simulink model "SVPWM"  (R2019a)
settings: Solver=FixedStepAuto  StartTime=0.0  StopTime=.1  FixedStep=1e-6  RelTol=1e-3
libraries: powerlib x8
settings Model: Creator=sange  LastModifiedBy=sange

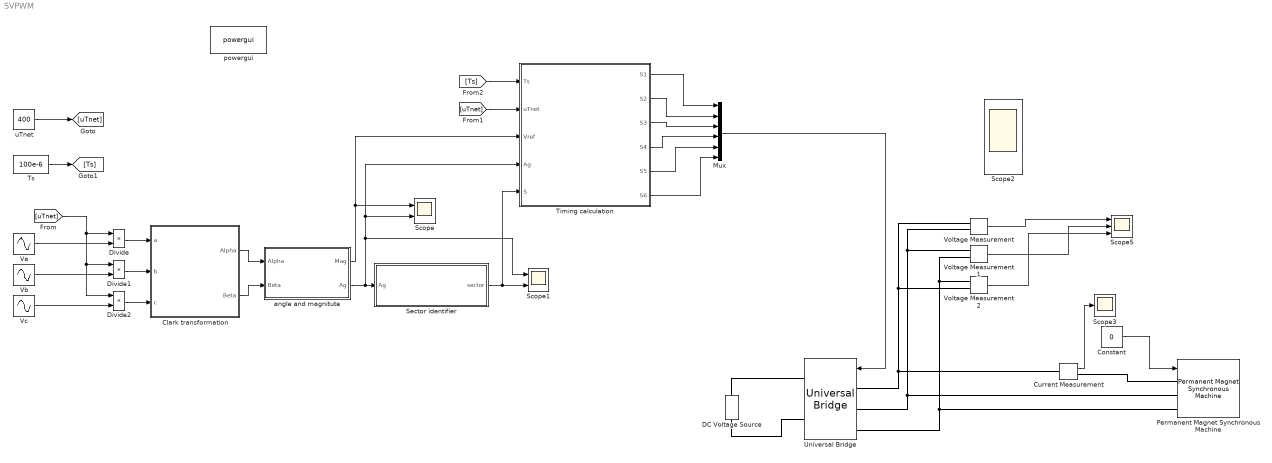
== system SVPWM ==
  Clark transformation : Subsystem
  Constant : Constant  Value=0
  Current Measurement : powerlib/Measurements/Current Measurement  PhasorSimulation=off  OutputType=Complex  PSBequivalent=0
      settings: SourceProductName=Simscape Electrical
  DC Voltage Source : powerlib/Electrical Sources/DC Voltage Source  Amplitude=400  Measurements=None
      settings: SourceProductName=Simscape Electrical
  Divide : Product  Inputs=**
  Divide1 : Product  Inputs=**
  Divide2 : Product  Inputs=**
  Mux : Mux  Inputs=6
  Permanent Magnet Synchronous Machine : powerlib/Machines/Permanent Magnet Synchronous Machine  NbPhases=3  FluxDistribution=Sinusoidal  RotorType=Round  MechanicalLoad=Torque Tm  PresetModel=No  ShowDetailedParameters=on  MeasurementBus=off  Resistance=0.0485  Inductance=8.5e-3  dqInductances=[8.5e-3,8.5e-3]  La=0.000395  MachineConstant=Flux linkage established by magnets (V.s)  Flux=0.1194  VoltageCst=86.6271  TorqueCst=0.7164  Flat=120  Mechanical=[0.0027 0.0004924 4 0]  PolePairs=4  InitialConditions=[0,0, 0,0]  InitialConditions5ph=[0 0 0 0 0 0]  TsPowergui=0  TsBlock=-1  RefAngle=Aligned with phase A axis (original Park)
  Scope : Scope  NumInputPorts=2
  Scope1 : Scope  NumInputPorts=2
  Scope2 : Scope  NumInputPorts=6
  Scope3 : Scope
  Scope5 : Scope  NumInputPorts=3
  Sector identifier : Subsystem
  "Timing calculation " : Subsystem
  "Ts " : Constant  Value=100e-6
  Universal Bridge : powerlib/Power Electronics/Universal Bridge  Arms=3  SnubberResistance=1e5  SnubberCapacitance=inf  Device=MOSFET / Diodes  Ron=1e-3  Lon=0  ForwardVoltages="[  0  0  ]"  ForwardVoltage=0  GTOparameters=[ 10e-6 , 20e-6 ]  IGBTparameters=[ 1e-6 , 2e-6 ]  Measurements=None  Measurements_2=None  converterType=Rectifier
      settings: SourceProductName=Simscape Electrical
  Va : Sin  Frequency=2*pi*100  SampleTime=0
  Vb : Sin  Frequency=2*pi*0100  Phase=-2*(pi/3)  SampleTime=0
  Vc : Sin  Frequency=2*pi*100  Phase=-4*(pi/3)  SampleTime=0
  Voltage Measurement : powerlib/Measurements/Voltage Measurement  PhasorSimulation=off  OutputType=Complex  PSBequivalent=0
      settings: SourceProductName=Simscape Electrical
  Voltage Measurement1 : powerlib/Measurements/Voltage Measurement  PhasorSimulation=off  OutputType=Complex  PSBequivalent=0
      settings: SourceProductName=Simscape Electrical
  Voltage Measurement2 : powerlib/Measurements/Voltage Measurement  PhasorSimulation=off  OutputType=Complex  PSBequivalent=0
      settings: SourceProductName=Simscape Electrical
  angle and magnitute : Subsystem
  powergui : powerlib/powergui  Priority=1  SimulationMode=Continuous  SampleTime=50e-6  frequency=60  Iterations=50  frequencyindice=0  Pbase=100e6  ErrMax=1e-4  UnitsV=kV  UnitsW=MW  buscounter=0  FunctionMessages=off  echomessages=off  EnableUseOfTLC=off  CurrentSourceSwitches=off  DisableSnubberDevices=off  DisableRonSwitches=off  DisableVfSwitches=off  DisplayEquations=off  AutomaticDiscreteSolvers=off  SolverType=Tustin/Backward Euler (TBE)  Interpol=off  ExternalGateDelay=off  methode=off  Ts=100  x0status=blocks  SPID=on  SwTol=0  HookPort=off  NonlinearTolerance=0  nMaxIteration=15  ContinueOnMaxIteration=off  RestoreLinks=warning  ResistiveCurrentMeasurement=off  Frange=[0:2:500]  Ylog=off  Xlog=on  ShowGrid=off  save=off  variable=ZData  structure=0  ZoomFFT=off  StartTime=0.0  cycles=1  DisplayStyle=1  fundamental=60  FreqAxis=off  MaxFrequency=1000  frequencyindicesteady=1  RmsSteady=1  display=off
      settings: SourceProductName=Simscape Electrical
  uTnet : Constant  Value=400
  wires:
  Clark transformation/1(Alpha) -> angle and magnitute/1(Alpha)
  Clark transformation/2(Beta) -> angle and magnitute/2(Beta)
  angle and magnitute/2(Ag) -> "Timing calculation "/4(Ag), Scope/2, Scope1/1, Sector identifier/1(Ag)
  Sector identifier/1(sector) -> "Timing calculation "/5(S), Scope1/2
  uTnet/1 -> [uTnet]
  Divide1/1 -> Clark transformation/2(b)
  Divide/1 -> Clark transformation/1(a)
  Divide2/1 -> Clark transformation/3(c)
  [uTnet] -> Divide1/1, Divide2/1, Divide/1
  Va/1 -> Divide/2
  Vb/1 -> Divide1/2
  Vc/1 -> Divide2/2
  "Ts "/1 -> [Ts]
  angle and magnitute/1(Mag) -> "Timing calculation "/3(Vref), Scope/1
  [uTnet] -> "Timing calculation "/2(uTnet)
  [Ts] -> "Timing calculation "/1(Ts)
  "Timing calculation "/1(S1) -> Mux/1
  "Timing calculation "/6(S6) -> Mux/6
  Mux/1 -> Universal Bridge/1
  Voltage Measurement/1 -> Scope5/1
  Voltage Measurement1/1 -> Scope5/2
  Voltage Measurement2/1 -> Scope5/3
  Current Measurement/1 -> Scope3/1
  Constant/1 -> Permanent Magnet Synchronous Machine/1
  "Timing calculation "/5("S5 ") -> Mux/5
  "Timing calculation "/4(S4) -> Mux/4
  "Timing calculation "/3("S3 ") -> Mux/3
  "Timing calculation "/2(S2) -> Mux/2
  connections:
  Voltage Measurement/LConn1 -- Universal Bridge/LConn1 -- Current Measurement/LConn1 -- Voltage Measurement2/LConn2
  DC Voltage Source/RConn1 -- Universal Bridge/RConn1
  DC Voltage Source/LConn1 -- Universal Bridge/RConn2
  Universal Bridge/LConn2 -- Permanent Magnet Synchronous Machine/LConn2 -- Voltage Measurement1/LConn1 -- Voltage Measurement/LConn2
  Universal Bridge/LConn3 -- Permanent Magnet Synchronous Machine/LConn3 -- Voltage Measurement1/LConn2 -- Voltage Measurement2/LConn1
  Current Measurement/RConn1 -- Permanent Magnet Synchronous Machine/LConn1

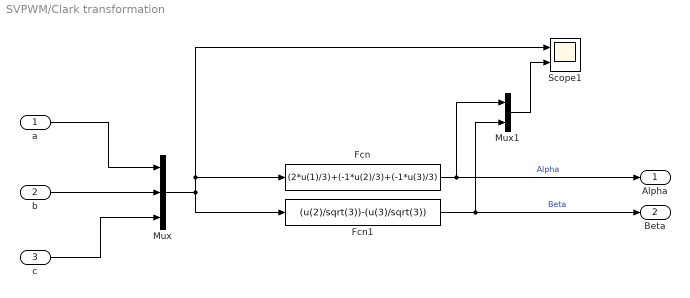
== system SVPWM/Clark transformation ==
  a : Inport
  b : Inport  Port=2
  c : Inport  Port=3
  Fcn : Fcn  Expr=(2*u(1)/3)+(-1*u(2)/3)+(-1*u(3)/3)
  Fcn1 : Fcn  Expr=(u(2)/sqrt(3))-(u(3)/sqrt(3))
  Mux : Mux  Inputs=3
  Mux1 : Mux  Inputs=2
  Scope1 : Scope  NumInputPorts=2
  Alpha : Outport
  Beta : Outport  Port=2
  wires:
  Mux/1 -> Scope1/1, Fcn/1, Fcn1/1
  Fcn1/1 -> Beta/1, Mux1/2  "Beta"
  c/1 -> Mux/3
  Fcn/1 -> Alpha/1, Mux1/1  "Alpha"
  a/1 -> Mux/1
  Mux1/1 -> Scope1/2
  b/1 -> Mux/2

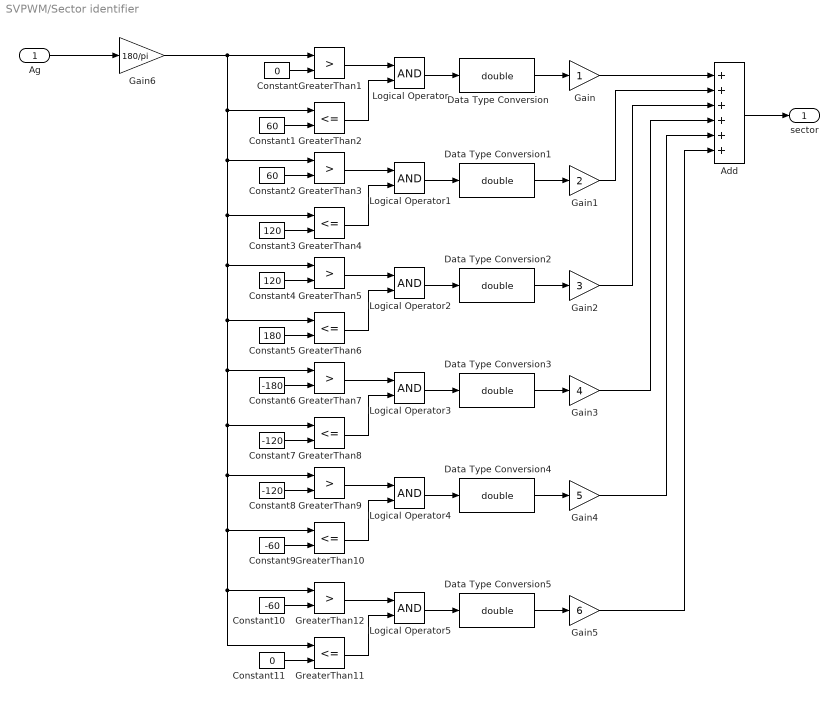
== system SVPWM/Sector identifier ==
  Ag : Inport
  Add : Sum  Inputs=++++++
  Constant : Constant  Value=0  OutDataTypeStr=double
  Constant1 : Constant  Value=60
  Constant10 : Constant  Value=-60
  Constant11 : Constant  Value=0
  Constant2 : Constant  Value=60
  Constant3 : Constant  Value=120
  Constant4 : Constant  Value=120
  Constant5 : Constant  Value=180
  Constant6 : Constant  Value=-180
  Constant7 : Constant  Value=-120
  Constant8 : Constant  Value=-120
  Constant9 : Constant  Value=-60
  Data Type Conversion{,1..5} (6 alike) : DataTypeConversion  OutDataTypeStr=double
  Gain : Gain
  Gain1 : Gain  Gain=2
  Gain2 : Gain  Gain=3
  Gain3 : Gain  Gain=4
  Gain4 : Gain  Gain=5
  Gain5 : Gain  Gain=6
  Gain6 : Gain  Gain=180/pi  OutDataTypeStr=double
  GreaterThan{1,3,5,7,9,12} (6 alike) : RelationalOperator  Operator=>  OutDataTypeStr=boolean  RndMeth=Simplest
  GreaterThan{2,4,6,8,10..11} (6 alike) : RelationalOperator  Operator=<=  OutDataTypeStr=boolean  RndMeth=Simplest
  Logical Operator{,1..5} (6 alike) : Logic  AllPortsSameDT=off  OutDataTypeStr=boolean
  sector : Outport
  wires:
  GreaterThan1/1 -> Logical Operator/1
  Constant/1 -> GreaterThan1/2
  Constant1/1 -> GreaterThan2/2
  GreaterThan2/1 -> Logical Operator/2
  Logical Operator/1 -> Data Type Conversion/1
  Data Type Conversion/1 -> Gain/1
  Gain/1 -> Add/1
  GreaterThan3/1 -> Logical Operator1/1
  Constant3/1 -> GreaterThan4/2
  Data Type Conversion1/1 -> Gain1/1
  Logical Operator1/1 -> Data Type Conversion1/1
  Gain1/1 -> Add/2
  Constant2/1 -> GreaterThan3/2
  GreaterThan4/1 -> Logical Operator1/2
  GreaterThan5/1 -> Logical Operator2/1
  Constant5/1 -> GreaterThan6/2
  Data Type Conversion2/1 -> Gain2/1
  Logical Operator2/1 -> Data Type Conversion2/1
  Gain2/1 -> Add/3
  Constant4/1 -> GreaterThan5/2
  GreaterThan6/1 -> Logical Operator2/2
  GreaterThan7/1 -> Logical Operator3/1
  Constant7/1 -> GreaterThan8/2
  Data Type Conversion3/1 -> Gain3/1
  Logical Operator3/1 -> Data Type Conversion3/1
  Gain3/1 -> Add/4
  Constant6/1 -> GreaterThan7/2
  GreaterThan8/1 -> Logical Operator3/2
  Gain4/1 -> Add/5
  GreaterThan10/1 -> Logical Operator4/2
  Data Type Conversion4/1 -> Gain4/1
  Constant9/1 -> GreaterThan10/2
  Constant8/1 -> GreaterThan9/2
  Logical Operator4/1 -> Data Type Conversion4/1
  GreaterThan9/1 -> Logical Operator4/1
  Logical Operator5/1 -> Data Type Conversion5/1
  Gain5/1 -> Add/6
  Constant10/1 -> GreaterThan12/2
  GreaterThan11/1 -> Logical Operator5/2
  GreaterThan12/1 -> Logical Operator5/1
  Data Type Conversion5/1 -> Gain5/1
  Constant11/1 -> GreaterThan11/2
  Add/1 -> sector/1
  Gain6/1 -> GreaterThan11/1, GreaterThan12/1, GreaterThan10/1, GreaterThan9/1, GreaterThan8/1, GreaterThan7/1, GreaterThan6/1, GreaterThan5/1, GreaterThan4/1, GreaterThan3/1, GreaterThan2/1, GreaterThan1/1
  Ag/1 -> Gain6/1

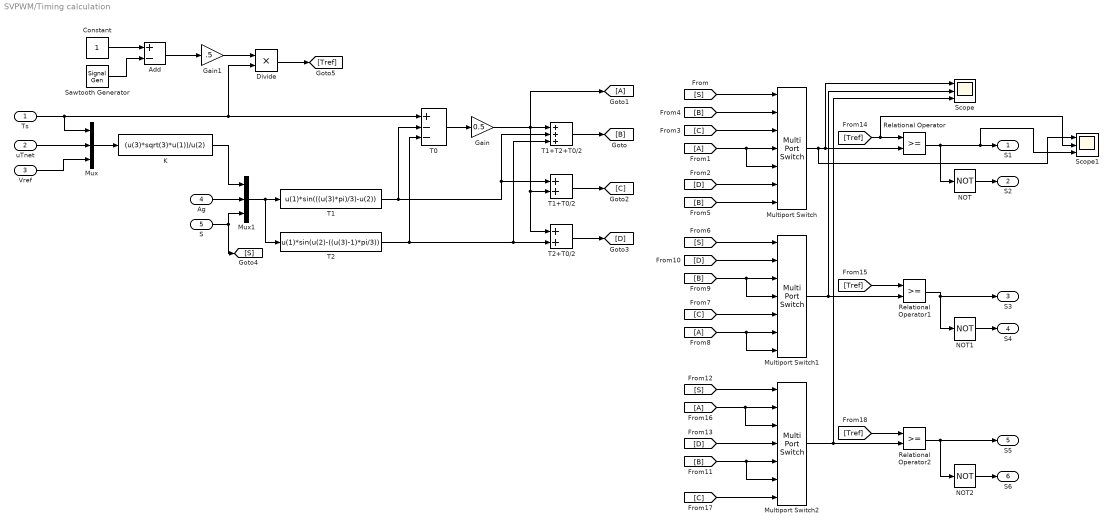
== system SVPWM/Timing calculation  ==
  Ts : Inport
  uTnet : Inport  Port=2
  Vref : Inport  Port=3
  Ag : Inport  Port=4
  S : Inport  Port=5
  Add : Sum  Inputs=+-
  Constant : Constant
  Divide : Product  Inputs=**
  Gain : Gain  Gain=0.5
  Gain1 : Gain  Gain=.5
  K : Fcn  Expr=(u(3)*sqrt(3)*u(1))/u(2)
  Multiport Switch : MultiPortSwitch  Inputs=6  DiagnosticForDefault=None
  Multiport Switch1 : MultiPortSwitch  Inputs=6  DiagnosticForDefault=None
  Multiport Switch2 : MultiPortSwitch  Inputs=6  DiagnosticForDefault=None
  Mux : Mux  Inputs=3
  Mux1 : Mux  Inputs=3
  NOT : Logic  Operator=NOT  IconShape=distinctive  AllPortsSameDT=off  OutDataTypeStr=boolean
  NOT1 : Logic  Operator=NOT  IconShape=distinctive  AllPortsSameDT=off  OutDataTypeStr=boolean
  NOT2 : Logic  Operator=NOT  IconShape=distinctive  AllPortsSameDT=off  OutDataTypeStr=boolean
  Relational Operator : RelationalOperator  OutDataTypeStr=boolean  RndMeth=Simplest
  Relational Operator1 : RelationalOperator  OutDataTypeStr=boolean  RndMeth=Simplest
  Relational Operator2 : RelationalOperator  OutDataTypeStr=boolean  RndMeth=Simplest
  Sawtooth Generator : SignalGenerator  WaveForm=sawtooth  Frequency=10000
  Scope : Scope  NumInputPorts=3
  Scope1 : Scope  NumInputPorts=3
  "T0 " : Sum  Inputs=+--
  T1 : Fcn  Expr=u(1)*sin(((u(3)*pi)/3)-u(2))
  T1+T0/2 : Sum
  T1+T2+T0/2 : Sum  Inputs=+++
  T2 : Fcn  Expr=u(1)*sin(u(2)-((u(3)-1)*pi/3))
  T2+T0/2 : Sum
  S1 : Outport
  S2 : Outport  Port=2
  "S3 " : Outport  Port=3
  S4 : Outport  Port=4
  "S5 " : Outport  Port=5
  S6 : Outport  Port=6
  wires:
  T2/1 -> T2+T0/2/2, T1+T2+T0/2/3, "T0 "/3
  Ts/1 -> Mux/1, Divide/2, "T0 "/1
  Mux/1 -> K/1
  uTnet/1 -> Mux/2
  K/1 -> Mux1/1
  Vref/1 -> Mux/3
  Mux1/1 -> T2/1, T1/1
  T1/1 -> T1+T0/2/1, T1+T2+T0/2/2, "T0 "/2
  S/1 -> [S], Mux1/3
  Ag/1 -> Mux1/2
  "T0 "/1 -> Gain/1
  Gain/1 -> [A], T2+T0/2/1, T1+T0/2/2, T1+T2+T0/2/1
  T1+T2+T0/2/1 -> [B]
  T1+T0/2/1 -> [C]
  T2+T0/2/1 -> [D]
  [S] -> Multiport Switch/1
  [B] -> Multiport Switch/2
  [C] -> Multiport Switch/3
  [A] -> Multiport Switch/5, Multiport Switch/4
  [D] -> Multiport Switch/6
  [B] -> Multiport Switch/7
  [S] -> Multiport Switch1/1
  [B] -> Multiport Switch1/4, Multiport Switch1/3
  [D] -> Multiport Switch1/2
  [A] -> Multiport Switch1/7, Multiport Switch1/6
  [S] -> Multiport Switch2/1
  [D] -> Multiport Switch2/4
  [A] -> Multiport Switch2/3, Multiport Switch2/2
  [C] -> Multiport Switch2/7
  [C] -> Multiport Switch1/5
  [B] -> Multiport Switch2/6, Multiport Switch2/5
  Sawtooth Generator/1 -> Add/2
  Constant/1 -> Add/1
  Add/1 -> Gain1/1
  Gain1/1 -> Divide/1
  Divide/1 -> [Tref]
  [Tref] -> Relational Operator/1, Scope1/2
  Multiport Switch/1 -> Scope1/1, Relational Operator/2, Scope/1
  Relational Operator/1 -> NOT/1, Scope1/3, S1/1
  NOT/1 -> S2/1
  Multiport Switch1/1 -> Relational Operator1/2, Scope/2
  Relational Operator1/1 -> "S3 "/1, NOT1/1
  NOT1/1 -> S4/1
  NOT2/1 -> S6/1
  Relational Operator2/1 -> NOT2/1, "S5 "/1
  Multiport Switch2/1 -> Relational Operator2/2, Scope/3
  [Tref] -> Relational Operator1/1
  [Tref] -> Relational Operator2/1

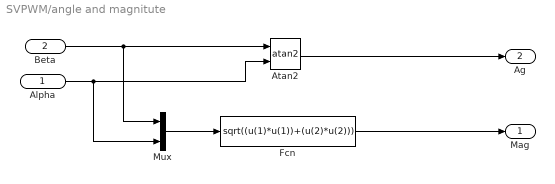
== system SVPWM/angle and magnitute ==
  Alpha : Inport
  Beta : Inport  Port=2
  Atan2 : Trigonometry  Operator=atan2
  Fcn : Fcn  Expr=sqrt((u(1)*u(1))+(u(2)*u(2)))
  Mux : Mux  Inputs=2
  Mag : Outport
  Ag : Outport  Port=2
  wires:
  Alpha/1 -> Atan2/2, Mux/2
  Fcn/1 -> Mag/1
  Beta/1 -> Atan2/1, Mux/1
  Mux/1 -> Fcn/1
  Atan2/1 -> Ag/1
